simulink model "FINAL_CSD_5LEVEL_SPWM_FIXED_DC_2"  (R2014a)
settings: Solver=ode45  StartTime=0.02  StopTime=0.4  RelTol=1e-3
libraries: powerlib x24, simulink x4
settings Model: Creator=PRAKASH BABU  LastModifiedBy=PRAKASH BABU

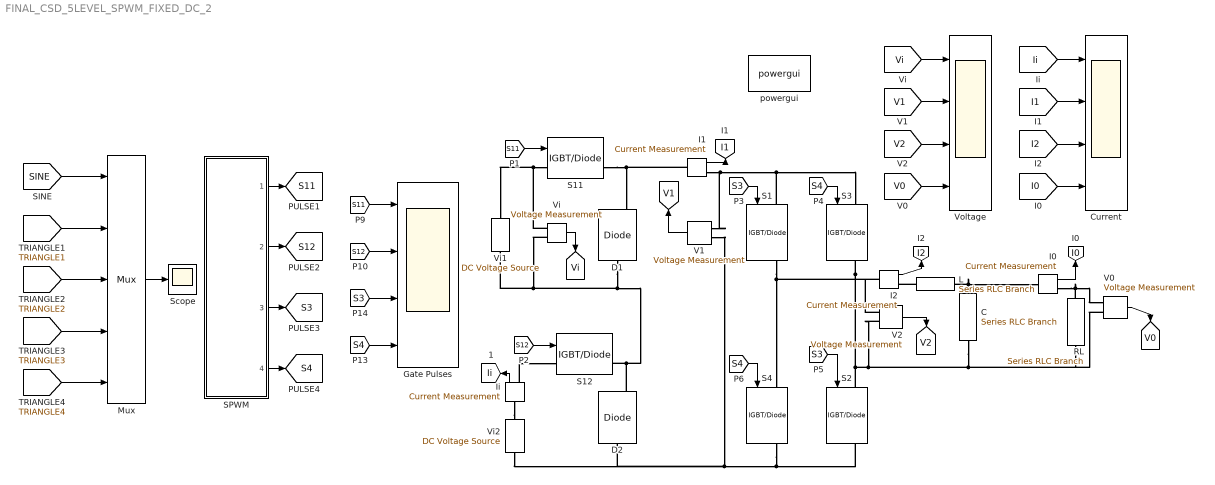
== system FINAL_CSD_5LEVEL_SPWM_FIXED_DC_2 ==
  C : powerlib/Elements/Series RLC Branch  LConnTagsString=__new0  RConnTagsString=__new0  BranchType=C  Resistance=1  Inductance=0.1  SetiL0=off  InitialCurrent=0  Capacitance=7e-6  Setx0=off  InitialVoltage=0  Measurements=None
  Current : Scope  NumInputPorts=4
      settings: YMin=0~-5~-5~-5  YMax=130~5~5~5  SaveName=current
  D1 : powerlib/Power Electronics/Diode  Ron=0.001  Lon=0  Vf=0.8  IC=0  UseSnubber=off  Rs=500  Cs=250e-9  Measurements=on
  D2 : powerlib/Power Electronics/Diode  Ron=0.001  Lon=0  Vf=0.8  IC=0  UseSnubber=off  Rs=500  Cs=250e-9  Measurements=on
  Gate Pulses : Scope  NumInputPorts=4
      settings: TimeRange=0.08  YMin=0~0~0~0  YMax=1~1~1~1  SaveName=gate
  I0 : powerlib/Measurements/Current Measurement  PhasorSimulation=off  OutputType=Complex  PSBequivalent=0
  I1 : powerlib/Measurements/Current Measurement  PhasorSimulation=off  OutputType=Complex  PSBequivalent=0
  I2 : powerlib/Measurements/Current Measurement  PhasorSimulation=off  OutputType=Complex  PSBequivalent=0
  Ii : powerlib/Measurements/Current Measurement  PhasorSimulation=off  OutputType=Complex  PSBequivalent=0
  L : powerlib/Elements/Series RLC Branch  LConnTagsString=__new0  RConnTagsString=__new0  BranchType=L  Resistance=1  Inductance=65e-3  SetiL0=off  InitialCurrent=0  Capacitance=1e-6  Setx0=off  InitialVoltage=0  Measurements=None
  Mux : Mux  Inputs=5
  RL : powerlib/Elements/Series RLC Branch  LConnTagsString=__new0  RConnTagsString=__new0  BranchType=R  Resistance=90  Inductance=10e-6  SetiL0=off  InitialCurrent=0  Capacitance=1e-6  Setx0=off  InitialVoltage=0  Measurements=None
  S{1..4,11..12} (6 alike) : powerlib/Power Electronics/IGBT//Diode  Ron=1e-3  Rs=1e5  Cs=inf  Measurements=on
  SPWM : Subsystem
  Scope : Scope
      settings: SaveName=sine
  V0 : powerlib/Measurements/Voltage Measurement  PhasorSimulation=off  OutputType=Complex  PSBequivalent=0
  V1 : powerlib/Measurements/Voltage Measurement  PhasorSimulation=off  OutputType=Complex  PSBequivalent=0
  V2 : powerlib/Measurements/Voltage Measurement  PhasorSimulation=off  OutputType=Complex  PSBequivalent=0
  Vi : powerlib/Measurements/Voltage Measurement  PhasorSimulation=off  OutputType=Complex  PSBequivalent=0
  Vi1 : powerlib/Electrical Sources/DC Voltage Source  Amplitude=115  Measurements=None
  Vi2 : powerlib/Electrical Sources/DC Voltage Source  Amplitude=115  Measurements=None
  Voltage : Scope  NumInputPorts=4
      settings: YMin=0~-5~-5~-5  YMax=130~5~5~5  SaveName=voltage
  powergui : powerlib/powergui  Priority=1  SimulationMode=Discrete  SolverType=Tustin  SampleTime=50e-6  frequency=60  SPID=off  DisableSnubberDevices=off  DisableRonSwitches=off  DisableVfSwitches=off  SwTol=0  Interpol=off  DisplayEquations=off  Ts=0  methode=off  frequencyindice=0  Pbase=100e6  ErrMax=1e-4  Iterations=50  UnitsV=kV  UnitsW=MW  FunctionMessages=off  echomessages=off  HookPort=off  EnableUseOfTLC=off  x0status=blocks  RestoreLinks=warning  ResistiveCurrentMeasurement=off  Frange=[0:2:500]  Ylog=off  Xlog=on  ShowGrid=off  save=off  variable=ZData  structure=voltage  ZoomFFT=off  StartTime=0.04  cycles=1  DisplayStyle=1  fundamental=50  FreqAxis=off  MaxFrequency=1000  frequencyindicesteady=1  RmsSteady=1  display=off
  tag scope: I0=global, I1=global, I2=global, Ii=global, S11=global, S12=global, S3=global, S4=global, V0=global, V1=global, V2=global, Vi=global
  wires:
  [SINE] -> Mux/1
  [TRIANGLE1] -> Mux/2
  [TRIANGLE2] -> Mux/3
  [TRIANGLE3] -> Mux/4
  [TRIANGLE4] -> Mux/5
  Mux/1 -> Scope/1
  [S11] -> Gate Pulses/1
  [S12] -> Gate Pulses/2
  [S3] -> Gate Pulses/3
  [S4] -> Gate Pulses/4
  V0/1 -> [V0]
  SPWM/1(1) -> [S11]
  SPWM/2(2) -> [S12]
  SPWM/3(3) -> [S3]
  SPWM/4(4) -> [S4]
  [S11] -> S11/1
  [S12] -> S12/1
  [S4] -> S3/1
  [S3] -> S1/1
  [S4] -> S4/1
  [S3] -> S2/1
  V1/1 -> [V1]
  V2/1 -> [V2]
  Vi/1 -> [Vi]
  [V1] -> Voltage/2
  [V2] -> Voltage/3
  [V0] -> Voltage/4
  [Vi] -> Voltage/1
  Ii/1 -> [Ii]
  I1/1 -> [I1]
  I0/1 -> [I0]
  I2/1 -> [I2]
  [I1] -> Current/2
  [I2] -> Current/3
  [I0] -> Current/4
  [Ii] -> Current/1
  connections:
  S4/RConn1 -- Vi2/LConn1 -- D2/LConn1 -- V1/LConn2 -- S2/RConn1
  S3/RConn1 -- V2/LConn2 -- V0/LConn2 -- RL/RConn1 -- C/RConn1 -- S2/LConn1
  D1/LConn1 -- Vi1/LConn1 -- Vi/LConn2 -- D2/RConn1 -- S12/RConn1
  V1/LConn1 -- I1/RConn1 -- S3/LConn1 -- S1/LConn1
  S1/RConn1 -- I2/LConn1 -- V2/LConn1 -- S4/LConn1
  Vi/LConn1 -- Vi1/RConn1 -- S11/LConn1
  Ii/LConn1 -- Vi2/RConn1
  Ii/RConn1 -- S12/LConn1
  S11/RConn1 -- I1/LConn1 -- D1/RConn1
  L/RConn1 -- I2/RConn1
  RL/LConn1 -- V0/LConn1 -- I0/RConn1
  C/LConn1 -- I0/LConn1 -- L/LConn1

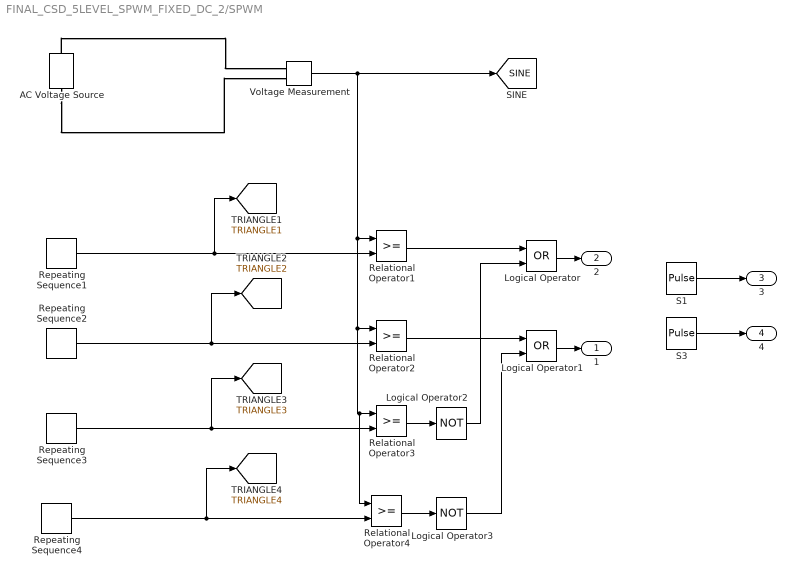
== system FINAL_CSD_5LEVEL_SPWM_FIXED_DC_2/SPWM ==
  AC Voltage Source : powerlib/Electrical Sources/AC Voltage Source  Amplitude=2  Phase=0  Frequency=50  SampleTime=0  Measurements=None
  Logical Operator : Logic  Operator=OR  AllPortsSameDT=off  OutDataTypeStr=boolean
  Logical Operator1 : Logic  Operator=OR  AllPortsSameDT=off  OutDataTypeStr=boolean
  Logical Operator2 : Logic  Operator=NOT  AllPortsSameDT=off  OutDataTypeStr=boolean
  Logical Operator3 : Logic  Operator=NOT  AllPortsSameDT=off  OutDataTypeStr=boolean
  Relational Operator{1..4} (4 alike) : RelationalOperator  OutDataTypeStr=boolean
  Repeating Sequence1 : simulink/Sources/Repeating Sequence  rep_seq_t=[0 0.5 1]/2500  rep_seq_y=[1 2 1]
  Repeating Sequence2 : simulink/Sources/Repeating Sequence  rep_seq_t=[0 0.5 1]/2500  rep_seq_y=[0 1 0]
  Repeating Sequence3 : simulink/Sources/Repeating Sequence  rep_seq_t=[0 0.5 1]/2500  rep_seq_y=[-1 0 -1]
  Repeating Sequence4 : simulink/Sources/Repeating Sequence  rep_seq_t=[0 0.5 1]/2500  rep_seq_y=[-2 -1 -2]
  S1 : DiscretePulseGenerator  PulseType=Time based  Period=0.02  PulseWidth=50
  S3 : DiscretePulseGenerator  PulseType=Time based  Period=0.02  PulseWidth=50  PhaseDelay=0.01
  Voltage Measurement : powerlib/Measurements/Voltage Measurement  PhasorSimulation=off  OutputType=Complex  PSBequivalent=0
  1 : Outport
  2 : Outport  Port=2
  3 : Outport  Port=3
  4 : Outport  Port=4
  tag scope: SINE=global, TRIANGLE1=global, TRIANGLE2=global, TRIANGLE3=global, TRIANGLE4=global
  wires:
  Repeating Sequence2/1 -> [TRIANGLE2], Relational Operator2/2
  Repeating Sequence1/1 -> [TRIANGLE1], Relational Operator1/2
  S1/1 -> 3/1
  S3/1 -> 4/1
  Repeating Sequence3/1 -> Relational Operator3/2, [TRIANGLE3]
  Voltage Measurement/1 -> Relational Operator4/1, Relational Operator3/1, Relational Operator2/1, Relational Operator1/1, [SINE]
  Repeating Sequence4/1 -> [TRIANGLE4], Relational Operator4/2
  Relational Operator3/1 -> Logical Operator2/1
  Relational Operator4/1 -> Logical Operator3/1
  Logical Operator1/1 -> 1/1
  Logical Operator/1 -> 2/1
  Relational Operator1/1 -> Logical Operator/1
  Logical Operator2/1 -> Logical Operator/2
  Relational Operator2/1 -> Logical Operator1/1
  Logical Operator3/1 -> Logical Operator1/2
  connections:
  AC Voltage Source/LConn1 -- Voltage Measurement/LConn2
  AC Voltage Source/RConn1 -- Voltage Measurement/LConn1
